simulink model "MassSpringDamper_trial"  (R2021a)
settings: Solver=VariableStepAuto  StartTime=0.0  StopTime=sim_time  RelTol=1e-3
values from neighbouring files (symbols this model uses):
  b = 3.5077E-6    (= 3.5077e-06)    [DCMotor_reduction_run.m]    (also in DCMotor_run.m; MassSpringDamper_run.m = 2; PID_ScriptOnly.m = 50; PID_SpringDamper_run.m = 10)
  F = 1    [MassSpringDamper_run.m]    (also in PID_SpringDamper_run.m = 10; TrainSimulation_run.m; TransferFunctionModel_run.m = 10)
  k = 20    [MassSpringDamper_run.m]    (also in PID_SpringDamper_run.m; PID_block_run.m; TrainSimulation_run.m = 1; TransferFunctionModel_run.m)
  M = 1    [MassSpringDamper_run.m]    (also in PID_SpringDamper_run.m; PID_block_run.m; PID_vehicle_run.m; TransferFunctionModel_run.m)
settings Model: Creator=shinyh  LastModifiedBy=shinyh
settings DataIOCC: Refine=250

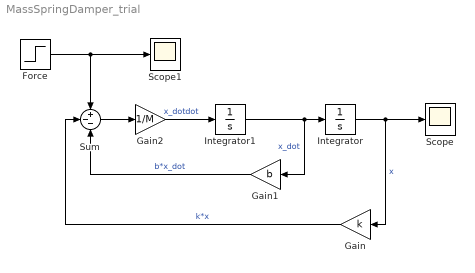
== system MassSpringDamper_trial ==
  Force : Step  After=F  SampleTime=0
  Gain : Gain  Gain=k
  Gain1 : Gain  Gain=b
  Gain2 : Gain  Gain=1/M
  Integrator : Integrator
  Integrator1 : Integrator
  Scope : Scope
  Scope1 : Scope
  Sum : Sum  Inputs=+--
  wires:
  Integrator/1 -> Scope/1, Gain/1  "x"
  Integrator1/1 -> Gain1/1, Integrator/1  "x_dot"
  Gain2/1 -> Integrator1/1  "x_dotdot"
  Gain/1 -> Sum/2  "k*x"
  Gain1/1 -> Sum/3  "b*x_dot"
  Force/1 -> Scope1/1, Sum/1
  Sum/1 -> Gain2/1
